simulink model "sim06c"  (R2020a)
settings: Solver=VariableStepAuto  StartTime=0.0  StopTime=10.0  RelTol=1e-3
values from neighbouring files (symbols this model uses):
  A = [-a1/A1,a1/A1;a1/A2,(-a1-a2)/A2]    [lab06.m]
  B = [1/A1,0;0,1/A2]    [lab06.m]
  C = [1,0;0,1]    [lab06.m]
  czas_skoku = 15    [lab06.m]
  D = [0,0;0,0]    [lab06.m]
  du1 = 0    [lab06.m]
  du2 = 0.1*fwe1max    (= 0.5)    [lab06.m]
  fwe1 = Tab_fwe1(i)    [lab06.m]
  fwe2 = 0.1*fwe1max    (= 0.5)    [lab06.m]
settings Model: Creator=jakub  LastModifiedBy=jakub

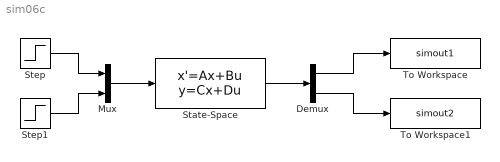
== system sim06c ==
  Demux : Demux  Outputs=2
  Mux : Mux  Inputs=2
  State-Space : StateSpace  A=A  B=B  C=C  D=D  InitialCondition=-A^(-1)*B*u
  Step : Step  Time=czas_skoku  Before=fwe1  After=fwe1 + du1  SampleTime=0
  Step1 : Step  Time=czas_skoku  Before=fwe2  After=fwe2 + du2  SampleTime=0
  To Workspace : ToWorkspace  VariableName=simout1  SampleTime=-1
  To Workspace1 : ToWorkspace  VariableName=simout2  SampleTime=-1
  wires:
  Mux/1 -> State-Space/1
  Step1/1 -> Mux/2
  Step/1 -> Mux/1
  State-Space/1 -> Demux/1
  Demux/1 -> To Workspace/1
  Demux/2 -> To Workspace1/1
